simulink model "disturb"  (R2016a)
settings: Solver=VariableStepAuto  StartTime=0.0  StopTime=40  RelTol=1e-3
settings Model: Creator=xin  LastModifiedBy=FWR

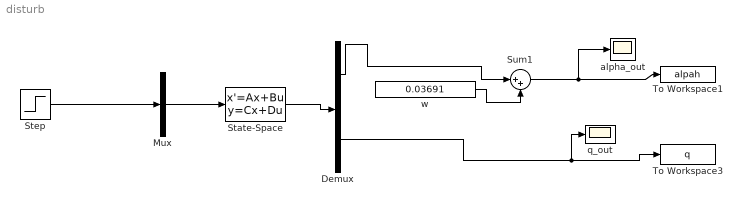
== system disturb ==
  Demux : Demux  Outputs=2
  Mux : Mux  Inputs=1
  State-Space : StateSpace  A=|  B=|  C=[0 57.29578 0 0;0 0 0 57.29578;]  D=[0; 0]  X0=[153 0.03691 0.03691 0]
      A=|
      | [-0.01931	8.8158	-32.17	-0.575;
      | -0.00025	-1.0189	0	-0.9051;
      | 0	0	0	1;
      | 0	0.822	0	-1.0774]
      B=|
      | [0.17370;
      | -0.00215
      | ;0;
      | -0.17555]
  Step : Step  Time=0  After=0.025  SampleTime=0
  Sum1 : Sum  Inputs=|++
  To Workspace1 : ToWorkspace  VariableName=alpah  SaveFormat=Timeseries  SampleTime=-1
  To Workspace3 : ToWorkspace  VariableName=q  SaveFormat=Timeseries  SampleTime=-1
  alpha_out : Scope
  q_out : Scope
  w : Constant  Value=0.03691
  wires:
  Step/1 -> Mux/1
  Mux/1 -> State-Space/1
  State-Space/1 -> Demux/1
  Demux/1 -> Sum1/1
  w/1 -> Sum1/2
  Sum1/1 -> To Workspace1/1, alpha_out/1
  Demux/2 -> q_out/1, To Workspace3/1
